simulink model "atrias_system"  (R2014a)
settings: Solver=FixedStepDiscrete  StartTime=0.0  StopTime=inf  FixedStep=sample_time  RelTol=1e-3
PreLoadFcn:
  | set_sampletime
PostLoadFcn:
  | set_sampletime
InitFcn:
  | sys_params
StartFcn:
  | set_sampletime
values from neighbouring files (symbols this model uses):
  A_lpf_velocity = 1 + B1_lpf_velocity + B2_lpf_velocity    [daq_params_osu.m]
  B1_lpf_velocity = -2*exp(-lpf_damping*fcut_velocity*sample_time)*cos(fcut_velocity*sample_time*sqrt(1-lpf_damping^2))    [daq_params_osu.m]
  B2_lpf_velocity = exp(-2*lpf_damping*fcut_velocity*sample_time)    [daq_params_osu.m]
  BOOM_MAX_ENCODER_TICKS = 2^17 - 1    (= 131071)    [daq_params_osu.m]
  BOOM_PITCH_CAL_VALUE_RAD = 0    [daq_params_osu.m]
  BOOM_PITCH_CAL_VALUE_TICKS = 43809    [daq_params_osu.m]
  BOOM_PITCH_ENCODER_RAD_PER_TICK = -2*pi / (2^17 * 2)    (= -2.39684498107e-05)    [daq_params_osu.m]
  BOOM_ROLL_CAL_VALUE_RAD = 0.1271    [daq_params_osu.m]
  BOOM_ROLL_CAL_VALUE_TICKS = 9318    [daq_params_osu.m]
  BOOM_ROLL_ENCODER_RAD_PER_TICK = 2*pi / (2^17 * 7)    (= 6.84812851735e-06)    [daq_params_osu.m]
  BOOM_YAW_ENCODER_RAD_PER_TICK = 2*pi / (2^17 * 9.6)    (= 4.9934270439e-06)    [daq_params_osu.m]
  CURRENT_LIMIT = 100    [daq_params_osu.m]
  fcut_smooth = 16*(2*pi)    (= 100.530964915)    [daq_params_osu.m]
  fcut_unwrap = 8*(2*pi)    (= 50.2654824574)    [daq_params_osu.m]
  gui_disable_cmd = 0    [daq_params_osu.m]
  gui_enable_cmd = 0    [daq_params_osu.m]
  gui_estop_cmd = 0    [daq_params_osu.m]
  gui_reset_cmd = 0    [daq_params_osu.m]
  HIP_ABS_ENCODER_RAD_PER_TICK = 2*pi / 2^13    (= 0.000766990393943)    [daq_params_osu.m]
  HIP_ABS_MAX_ENCODER_TICKS = 2^13 - 1    (= 8191)    [daq_params_osu.m]
  HIP_INC_ENCODER_RAD_PER_TICK = 2*pi / (2500 * 4 * 57)    (= 1.10231321179e-05)    [daq_params_osu.m]
  HIP_INC_MAX_ENCODER_TICKS = 2^16 - 1    (= 65535)    [daq_params_osu.m]
  HIP_MOTOR_CONSTANT = 0.184    [daq_params_osu.m]
  HIP_MTR_GEAR_RATIO = 57    [daq_params_osu.m]
  HIP_MTR_MAX_TORQUE = MTR_HIP_MAX_CURRENT*HIP_MOTOR_CONSTANT*HIP_MTR_GEAR_RATIO    (= 629.28)    [daq_params_osu.m]
  INC_ENC_DIRS = -[ LEG1_MOTOR_A_DIRECTION ... (first row only)    [daq_params_osu.m]
  INC_ENC_RAD_PER_TICK = 2*pi/14000/LEG_MTR_GEAR_RATIO    (= 8.97597901026e-06)    [daq_params_osu.m]
  k_sea = 4118    [sys_params.m]
  LEFT_HIP_CALIB_POS = 0    [daq_params_osu.m]
  LEFT_HIP_CALIB_VAL = 7192 - 2^13    (= -1000)    [daq_params_osu.m]
  LEFT_MOTOR_HIP_DIRECTION = -1.0    (= -1)    [daq_params_osu.m]
  LEG1_LEG_A_CALIB_VAL = 265635200    [daq_params_osu.m]
  LEG1_LEG_A_RAD_PER_CNT = -9.8039216e-09    [daq_params_osu.m]
  LEG1_LEG_B_CALIB_VAL = 174340930    [daq_params_osu.m]
  LEG1_LEG_B_RAD_PER_CNT = -9.8039216e-09    [daq_params_osu.m]
  LEG1_MOTOR_A_DIRECTION = -1.0    (= -1)    [daq_params_osu.m]
  LEG1_MOTOR_B_DIRECTION = -1.0    (= -1)    [daq_params_osu.m]
  LEG1_TRAN_A_CALIB_VAL = 142852340    [daq_params_osu.m]
  LEG1_TRAN_A_RAD_PER_CNT = 9.8039216e-09    [daq_params_osu.m]
  LEG1_TRAN_B_CALIB_VAL = 142241870    [daq_params_osu.m]
  LEG1_TRAN_B_RAD_PER_CNT = -9.8039216e-09    [daq_params_osu.m]
  LEG2_LEG_A_CALIB_VAL = 265322590    [daq_params_osu.m]
  LEG2_LEG_A_RAD_PER_CNT = -9.8039216e-09    [daq_params_osu.m]
  LEG2_LEG_B_CALIB_VAL = 261290850    [daq_params_osu.m]
  LEG2_LEG_B_RAD_PER_CNT = 9.8039216e-09    [daq_params_osu.m]
  LEG2_MOTOR_A_DIRECTION = 1.0    (= 1)    [daq_params_osu.m]
  LEG2_MOTOR_B_DIRECTION = 1.0    (= 1)    [daq_params_osu.m]
  LEG2_TRAN_A_CALIB_VAL = 142172760    [daq_params_osu.m]
  LEG2_TRAN_A_RAD_PER_CNT = 9.8039216e-09    [daq_params_osu.m]
  LEG2_TRAN_B_CALIB_VAL = 142444320    [daq_params_osu.m]
  LEG2_TRAN_B_RAD_PER_CNT = -9.8039216e-09    [daq_params_osu.m]
  LEG_A_CALIB_LOC = pi + 0.305432619099008    (= 3.44702527269)    [daq_params_osu.m]
  LEG_B_CALIB_LOC = pi - 0.305432619099008    (= 2.83616003449)    [daq_params_osu.m]
  LEG_MOTOR_CONSTANT = 0.119    [daq_params_osu.m]
  LEG_MTR_GEAR_RATIO = 50    [daq_params_osu.m]
  LEG_MTR_MAX_TORQUE = MTR_MAX_CURRENT*LEG_MOTOR_CONSTANT*LEG_MTR_GEAR_RATIO    (= 922.25)    [daq_params_osu.m]
  max_encoder_velocity = 200    [daq_params_osu.m]
  MEDULLA_ADC_MAX_VOLTS = 2.70    (= 2.7)    [daq_params_osu.m]
  MEDULLA_ADC_OFFSET_COUNTS = 172    [daq_params_osu.m]
  MEDULLA_STATE_ERROR = 5    [daq_params_osu.m]
  MEDULLA_STATE_HALT = 4    [daq_params_osu.m]
  MEDULLA_STATE_IDLE = 0    [daq_params_osu.m]
  MEDULLA_STATE_RESET = 6    [daq_params_osu.m]
  MEDULLA_STATE_RUN = 2    [daq_params_osu.m]
  MEDULLA_TIMER_FREQ = 32e6    (= 32000000)    [daq_params_osu.m]
  MOTOR_POSITION_LIMITS_LOWER = [2.5; 1.4; 0.4]    [daq_params_osu.m]
  MOTOR_POSITION_LIMITS_UPPER = [4.9; 3.8; 2.5]    [daq_params_osu.m]
  MTR_HIP_MAX_CURRENT = 60.0    (= 60)    [daq_params_osu.m]
  MTR_MAX_CONT_CURRENT = 100.0    (= 100)    [daq_params_osu.m]
  MTR_MAX_COUNT = 19900    [daq_params_osu.m]
  MTR_MAX_CURRENT = 155.0    (= 155)    [daq_params_osu.m]
  nom_sample_time = 0.001    [sys_params.m]
  RIGHT_HIP_CALIB_POS = 0    [daq_params_osu.m]
  RIGHT_HIP_CALIB_VAL = 1091    [daq_params_osu.m]
  RIGHT_MOTOR_HIP_DIRECTION = 1.0    (= 1)    [daq_params_osu.m]
  sample_time = 1/update_freq    (= 0.001)    [daq_params_osu.m]
  sensor_start_time = 8    [daq_params_osu.m]
undefined symbols (not defined in the file or in its folder): max_sensor_velocity
libraries: xpcethercatlib x194, simulink x50, slrtlib x2, dspswit3 x1
(part 2 of 4)

== system atrias_system/DAQ/Elmo Back Left ==
  MotorCmd : Inport
  Constant1 : Constant  Value=4  OutDataTypeStr=Inherit: Inherit via back propagation  SampleTime=-1
  Data Type Conversion124 : DataTypeConversion
  Data Type Conversion125 : DataTypeConversion
  Data Type Conversion126 : DataTypeConversion
  Data Type Conversion2 : DataTypeConversion  OutDataTypeStr=int16
  Drive state transition : Subsystem
  EtherCAT PDO Receive1 : xpcethercatlib/EtherCAT PDO Receive  Priority=2  sig_name=Drive 2 (Elmo Drive).Inputs.Status word  sig_offset=2928  sig_type=uint16  type_size=16  sig_dim=1  device_id=0  sample_time=0.001000
  EtherCAT PDO Receive2 : xpcethercatlib/EtherCAT PDO Receive  Priority=2  sig_name=Drive 2 (Elmo Drive).Inputs.Mode of operation display  sig_offset=2944  sig_type=int8  type_size=8  sig_dim=1  device_id=0  sample_time=0.001000
  "EtherCAT PDO Transmit " : xpcethercatlib/EtherCAT PDO Transmit   Priority=3  sig_name=Drive 2 (Elmo Drive).Outputs.Target Torque  sig_offset=2880  sig_type=int16  type_size=16  sig_dim=1  device_id=0  sample_time=0.001000
  EtherCAT PDO Transmit 1 : xpcethercatlib/EtherCAT PDO Transmit   Priority=3  sig_name=Drive 2 (Elmo Drive).Outputs.Control word  sig_offset=2896  sig_type=uint16  type_size=16  sig_dim=1  device_id=0  sample_time=0.001000
  EtherCAT PDO Transmit 2 : xpcethercatlib/EtherCAT PDO Transmit   Priority=3  sig_name=Drive 2 (Elmo Drive).Outputs.Mode of operation  sig_offset=2912  sig_type=int8  type_size=8  sig_dim=1  device_id=0  sample_time=0.001000
  Mux28 : Mux  Inputs=3
  status : Outport
  wires:
  EtherCAT PDO Receive1/1 -> Drive state transition/1(Status), Data Type Conversion126/1
  EtherCAT PDO Receive2/1 -> Data Type Conversion124/1
  Mux28/1 -> status/1
  Data Type Conversion126/1 -> Mux28/1  "Status Word"
  Data Type Conversion124/1 -> Mux28/2  "Mode of Operation"
  Constant1/1 -> Data Type Conversion125/1
  Drive state transition/1(Control) -> Mux28/3, EtherCAT PDO Transmit 1/1
  Data Type Conversion125/1 -> EtherCAT PDO Transmit 2/1
  MotorCmd/1 -> Data Type Conversion2/1
  Data Type Conversion2/1 -> "EtherCAT PDO Transmit "/1

== system atrias_system/DAQ/Elmo Back Right ==
  MotorCmd : Inport
  Constant1 : Constant  Value=4  OutDataTypeStr=Inherit: Inherit via back propagation  SampleTime=-1
  Data Type Conversion124 : DataTypeConversion
  Data Type Conversion125 : DataTypeConversion
  Data Type Conversion126 : DataTypeConversion
  Data Type Conversion2 : DataTypeConversion  OutDataTypeStr=int16
  Drive state transition : Subsystem
  EtherCAT PDO Receive1 : xpcethercatlib/EtherCAT PDO Receive  Priority=2  sig_name=Drive 9 (Elmo Drive).Inputs.Status word  sig_offset=3168  sig_type=uint16  type_size=16  sig_dim=1  device_id=0  sample_time=0.001000
  EtherCAT PDO Receive2 : xpcethercatlib/EtherCAT PDO Receive  Priority=2  sig_name=Drive 9 (Elmo Drive).Inputs.Mode of operation display  sig_offset=3184  sig_type=int8  type_size=8  sig_dim=1  device_id=0  sample_time=0.001000
  "EtherCAT PDO Transmit " : xpcethercatlib/EtherCAT PDO Transmit   Priority=3  sig_name=Drive 9 (Elmo Drive).Outputs.Target Torque  sig_offset=3120  sig_type=int16  type_size=16  sig_dim=1  device_id=0  sample_time=0.001000
  EtherCAT PDO Transmit 1 : xpcethercatlib/EtherCAT PDO Transmit   Priority=3  sig_name=Drive 9 (Elmo Drive).Outputs.Control word  sig_offset=3136  sig_type=uint16  type_size=16  sig_dim=1  device_id=0  sample_time=0.001000
  EtherCAT PDO Transmit 2 : xpcethercatlib/EtherCAT PDO Transmit   Priority=3  sig_name=Drive 9 (Elmo Drive).Outputs.Mode of operation  sig_offset=3152  sig_type=int8  type_size=8  sig_dim=1  device_id=0  sample_time=0.001000
  Mux28 : Mux  Inputs=3
  status : Outport
  wires:
  EtherCAT PDO Receive1/1 -> Drive state transition/1(Status), Data Type Conversion126/1
  EtherCAT PDO Receive2/1 -> Data Type Conversion124/1
  Mux28/1 -> status/1
  Data Type Conversion126/1 -> Mux28/1  "Status Word"
  Data Type Conversion124/1 -> Mux28/2  "Mode of Operation"
  Constant1/1 -> Data Type Conversion125/1
  Drive state transition/1(Control) -> Mux28/3, EtherCAT PDO Transmit 1/1
  Data Type Conversion125/1 -> EtherCAT PDO Transmit 2/1
  MotorCmd/1 -> Data Type Conversion2/1
  Data Type Conversion2/1 -> "EtherCAT PDO Transmit "/1

== system atrias_system/DAQ/Elmo Front Left ==
  MotorCmd : Inport
  Constant1 : Constant  Value=4  OutDataTypeStr=Inherit: Inherit via back propagation  SampleTime=-1
  Data Type Conversion124 : DataTypeConversion
  Data Type Conversion125 : DataTypeConversion
  Data Type Conversion126 : DataTypeConversion
  Data Type Conversion2 : DataTypeConversion  OutDataTypeStr=int16
  Drive state transition : Subsystem
  EtherCAT PDO Receive1 : xpcethercatlib/EtherCAT PDO Receive  Priority=2  sig_name=Drive 3 (Elmo Drive).Inputs.Status word  sig_offset=3008  sig_type=uint16  type_size=16  sig_dim=1  device_id=0  sample_time=0.001000
  EtherCAT PDO Receive2 : xpcethercatlib/EtherCAT PDO Receive  Priority=2  sig_name=Drive 3 (Elmo Drive).Inputs.Mode of operation display  sig_offset=3024  sig_type=int8  type_size=8  sig_dim=1  device_id=0  sample_time=0.001000
  "EtherCAT PDO Transmit " : xpcethercatlib/EtherCAT PDO Transmit   Priority=3  sig_name=Drive 3 (Elmo Drive).Outputs.Target Torque  sig_offset=2960  sig_type=int16  type_size=16  sig_dim=1  device_id=0  sample_time=0.001000
  EtherCAT PDO Transmit 1 : xpcethercatlib/EtherCAT PDO Transmit   Priority=3  sig_name=Drive 3 (Elmo Drive).Outputs.Control word  sig_offset=2976  sig_type=uint16  type_size=16  sig_dim=1  device_id=0  sample_time=0.001000
  EtherCAT PDO Transmit 2 : xpcethercatlib/EtherCAT PDO Transmit   Priority=3  sig_name=Drive 3 (Elmo Drive).Outputs.Mode of operation  sig_offset=2992  sig_type=int8  type_size=8  sig_dim=1  device_id=0  sample_time=0.001000
  Mux28 : Mux  Inputs=3
  status : Outport
  wires:
  EtherCAT PDO Receive1/1 -> Drive state transition/1(Status), Data Type Conversion126/1
  EtherCAT PDO Receive2/1 -> Data Type Conversion124/1
  Mux28/1 -> status/1
  Data Type Conversion126/1 -> Mux28/1  "Status Word"
  Data Type Conversion124/1 -> Mux28/2  "Mode of Operation"
  Constant1/1 -> Data Type Conversion125/1
  Drive state transition/1(Control) -> Mux28/3, EtherCAT PDO Transmit 1/1
  Data Type Conversion125/1 -> EtherCAT PDO Transmit 2/1
  MotorCmd/1 -> Data Type Conversion2/1
  Data Type Conversion2/1 -> "EtherCAT PDO Transmit "/1

== system atrias_system/DAQ/Elmo Front Right ==
  MotorCmd : Inport
  Constant1 : Constant  Value=4  OutDataTypeStr=Inherit: Inherit via back propagation  SampleTime=-1
  Data Type Conversion124 : DataTypeConversion
  Data Type Conversion125 : DataTypeConversion
  Data Type Conversion126 : DataTypeConversion
  Data Type Conversion2 : DataTypeConversion  OutDataTypeStr=int16
  Drive state transition : Subsystem
  EtherCAT PDO Receive1 : xpcethercatlib/EtherCAT PDO Receive  Priority=2  sig_name=Drive 8 (Elmo Drive).Inputs.Status word  sig_offset=3088  sig_type=uint16  type_size=16  sig_dim=1  device_id=0  sample_time=0.001000
  EtherCAT PDO Receive2 : xpcethercatlib/EtherCAT PDO Receive  Priority=2  sig_name=Drive 8 (Elmo Drive).Inputs.Mode of operation display  sig_offset=3104  sig_type=int8  type_size=8  sig_dim=1  device_id=0  sample_time=0.001000
  "EtherCAT PDO Transmit " : xpcethercatlib/EtherCAT PDO Transmit   Priority=3  sig_name=Drive 8 (Elmo Drive).Outputs.Target Torque  sig_offset=3040  sig_type=int16  type_size=16  sig_dim=1  device_id=0  sample_time=0.001000
  EtherCAT PDO Transmit 1 : xpcethercatlib/EtherCAT PDO Transmit   Priority=3  sig_name=Drive 8 (Elmo Drive).Outputs.Control word  sig_offset=3056  sig_type=uint16  type_size=16  sig_dim=1  device_id=0  sample_time=0.001000
  EtherCAT PDO Transmit 2 : xpcethercatlib/EtherCAT PDO Transmit   Priority=3  sig_name=Drive 8 (Elmo Drive).Outputs.Mode of operation  sig_offset=3072  sig_type=int8  type_size=8  sig_dim=1  device_id=0  sample_time=0.001000
  Mux28 : Mux  Inputs=3
  status : Outport
  wires:
  EtherCAT PDO Receive1/1 -> Drive state transition/1(Status), Data Type Conversion126/1
  EtherCAT PDO Receive2/1 -> Data Type Conversion124/1
  Mux28/1 -> status/1
  Data Type Conversion126/1 -> Mux28/1  "Status Word"
  Data Type Conversion124/1 -> Mux28/2  "Mode of Operation"
  Constant1/1 -> Data Type Conversion125/1
  Drive state transition/1(Control) -> Mux28/3, EtherCAT PDO Transmit 1/1
  Data Type Conversion125/1 -> EtherCAT PDO Transmit 2/1
  MotorCmd/1 -> Data Type Conversion2/1
  Data Type Conversion2/1 -> "EtherCAT PDO Transmit "/1

== system atrias_system/DAQ/Fail Safe ==
  note: any of the absolute leg encoders read zero?
  note: all encoders read zero?
  note: any of the absolute lateral encdoers read all
      | zeros/ones in the first 10 readings?
  encoder signals : Inport
  Clock : Clock
  Compare To Constant : simulink/Logic and Bit Operations/Compare To Constant  relop===  const=2^13-1  OutDataTypeStr=boolean
  Compare To Zero : simulink/Logic and Bit Operations/Compare To Zero  relop===  OutDataTypeStr=boolean
  Compare To Zero1 : simulink/Logic and Bit Operations/Compare To Zero  relop===  OutDataTypeStr=boolean
  Compare To Zero2 : simulink/Logic and Bit Operations/Compare To Zero  relop===  OutDataTypeStr=boolean
  Data Type Conversion : DataTypeConversion  OutDataTypeStr=boolean
  Data Type Conversion1 : DataTypeConversion  OutDataTypeStr=boolean
  Data Type Conversion2 : DataTypeConversion  OutDataTypeStr=uint8
  Data Type Conversion3 : DataTypeConversion  OutDataTypeStr=uint8
  Initial Sensor Reading : simulink/Logic and Bit Operations/Compare To Constant  relop=<=  const=sensor_start_time+10*sample_time  OutDataTypeStr=boolean
  Logical Operator{,1,3..4} (4 alike) : Logic  AllPortsSameDT=off  OutDataTypeStr=boolean
  Logical Operator2 : Logic  Operator=OR  Inputs=3  AllPortsSameDT=off  OutDataTypeStr=boolean
  LogicalOperator5 : Logic  Operator=OR  AllPortsSameDT=off  OutDataTypeStr=boolean
  Sensors Active : simulink/Logic and Bit Operations/Compare To Constant  relop=>=  const=sensor_start_time  OutDataTypeStr=boolean
  Sum of Elements : Sum  Inputs=+
  Sum of Elements1 : Sum  Inputs=+
  Sum of Elements2 : Sum  Inputs=+
  absolute lateral encoders : Selector  InputPortWidth=15  Indices=[9 11]
  absolute leg encoders : Selector  InputPortWidth=15  Indices=[1 2 3 4 5 6 7 8]
  stop? : Outport
  wires:
  LogicalOperator5/1 -> Logical Operator3/2
  Compare To Constant/1 -> LogicalOperator5/2
  Compare To Zero2/1 -> LogicalOperator5/1
  absolute leg encoders/1 -> Compare To Zero1/1
  Compare To Zero1/1 -> Logical Operator1/2
  Logical Operator2/1 -> stop?/1
  Logical Operator1/1 -> Data Type Conversion2/1
  Compare To Zero/1 -> Logical Operator/1
  encoder signals/1 -> absolute lateral encoders/1, absolute leg encoders/1, Sum of Elements/1
  Logical Operator/1 -> Logical Operator2/1
  Sum of Elements/1 -> Compare To Zero/1
  Sensors Active/1 -> Logical Operator4/1, Logical Operator/2, Logical Operator1/1
  absolute lateral encoders/1 -> Compare To Zero2/1, Compare To Constant/1
  Clock/1 -> Initial Sensor Reading/1, Sensors Active/1
  Initial Sensor Reading/1 -> Logical Operator4/2
  Logical Operator4/1 -> Logical Operator3/1
  Logical Operator3/1 -> Data Type Conversion3/1
  Sum of Elements1/1 -> Data Type Conversion/1
  Sum of Elements2/1 -> Data Type Conversion1/1
  Data Type Conversion/1 -> Logical Operator2/3
  Data Type Conversion1/1 -> Logical Operator2/2
  Data Type Conversion2/1 -> Sum of Elements2/1
  Data Type Conversion3/1 -> Sum of Elements1/1

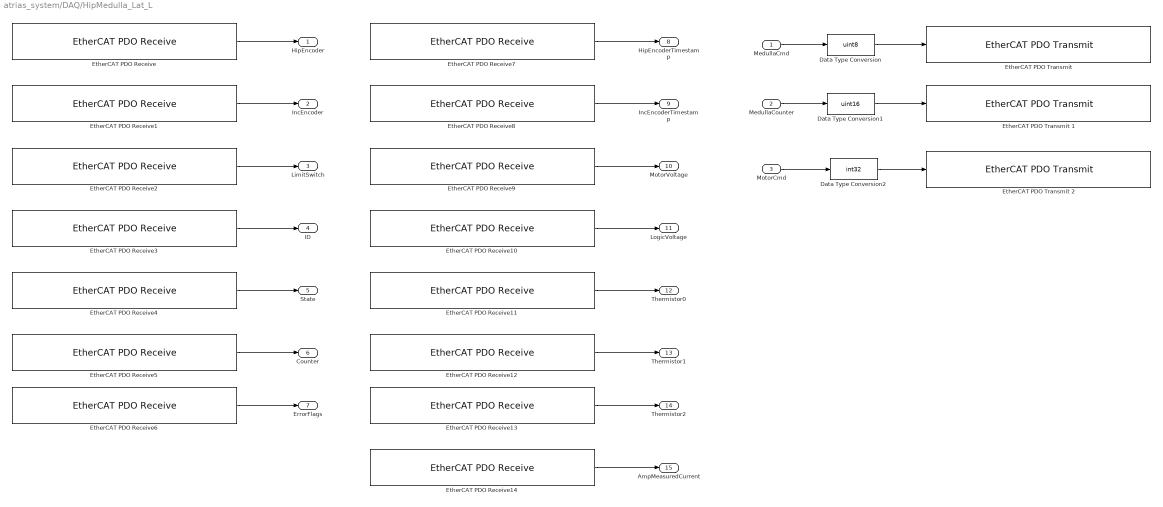
== system atrias_system/DAQ/HipMedulla_Lat_L ==
  MedullaCmd : Inport
  MedullaCounter : Inport  Port=2
  MotorCmd : Inport  Port=3
  Data Type Conversion : DataTypeConversion  OutDataTypeStr=uint8
  Data Type Conversion1 : DataTypeConversion  OutDataTypeStr=uint16
  Data Type Conversion2 : DataTypeConversion  OutDataTypeStr=int32
  EtherCAT PDO Receive : xpcethercatlib/EtherCAT PDO Receive  Priority=2  sig_name=Box 1 (ATRIAS 2.1 Hip (Medulla 1.5)).Hip Encoder.Encoder  sig_offset=632  sig_type=uint32  type_size=32  sig_dim=1  device_id=0  sample_time=0.001000
  EtherCAT PDO Receive1 : xpcethercatlib/EtherCAT PDO Receive  Priority=2  sig_name=Box 1 (ATRIAS 2.1 Hip (Medulla 1.5)).Incremental Encoder.Incremental Encoder  sig_offset=776  sig_type=uint16  type_size=16  sig_dim=1  device_id=0  sample_time=0.001000
  EtherCAT PDO Receive10 : xpcethercatlib/EtherCAT PDO Receive  Priority=2  sig_name=Box 1 (ATRIAS 2.1 Hip (Medulla 1.5)).Power.Logic Voltage  sig_offset=696  sig_type=uint16  type_size=16  sig_dim=1  device_id=0  sample_time=0.001000
  EtherCAT PDO Receive11 : xpcethercatlib/EtherCAT PDO Receive  Priority=2  sig_name=Box 1 (ATRIAS 2.1 Hip (Medulla 1.5)).Thermistors.Thermistor 0  sig_offset=712  sig_type=uint16  type_size=16  sig_dim=1  device_id=0  sample_time=0.001000
  EtherCAT PDO Receive12 : xpcethercatlib/EtherCAT PDO Receive  Priority=2  sig_name=Box 1 (ATRIAS 2.1 Hip (Medulla 1.5)).Thermistors.Thermistor 1  sig_offset=728  sig_type=uint16  type_size=16  sig_dim=1  device_id=0  sample_time=0.001000
  EtherCAT PDO Receive13 : xpcethercatlib/EtherCAT PDO Receive  Priority=2  sig_name=Box 1 (ATRIAS 2.1 Hip (Medulla 1.5)).Thermistors.Thermistor 2  sig_offset=744  sig_type=uint16  type_size=16  sig_dim=1  device_id=0  sample_time=0.001000
  EtherCAT PDO Receive14 : xpcethercatlib/EtherCAT PDO Receive  Priority=2  sig_name=Box 1 (ATRIAS 2.1 Hip (Medulla 1.5)).Measured Current.Amp Measured Current  sig_offset=760  sig_type=int16  type_size=16  sig_dim=1  device_id=0  sample_time=0.001000
  EtherCAT PDO Receive2 : xpcethercatlib/EtherCAT PDO Receive  Priority=2  sig_name=Box 1 (ATRIAS 2.1 Hip (Medulla 1.5)).uController Status.Limit Switch  sig_offset=624  sig_type=uint8  type_size=8  sig_dim=1  device_id=0  sample_time=0.001000
  EtherCAT PDO Receive3 : xpcethercatlib/EtherCAT PDO Receive  Priority=2  sig_name=Box 1 (ATRIAS 2.1 Hip (Medulla 1.5)).uController Status.ID  sig_offset=592  sig_type=uint8  type_size=8  sig_dim=1  device_id=0  sample_time=0.001000
  EtherCAT PDO Receive4 : xpcethercatlib/EtherCAT PDO Receive  Priority=2  sig_name=Box 1 (ATRIAS 2.1 Hip (Medulla 1.5)).uController Status.State  sig_offset=600  sig_type=uint8  type_size=8  sig_dim=1  device_id=0  sample_time=0.001000
  EtherCAT PDO Receive5 : xpcethercatlib/EtherCAT PDO Receive  Priority=2  sig_name=Box 1 (ATRIAS 2.1 Hip (Medulla 1.5)).uController Status.Counter  sig_offset=608  sig_type=uint8  type_size=8  sig_dim=1  device_id=0  sample_time=0.001000
  EtherCAT PDO Receive6 : xpcethercatlib/EtherCAT PDO Receive  Priority=2  sig_name=Box 1 (ATRIAS 2.1 Hip (Medulla 1.5)).uController Status.Error Flags  sig_offset=616  sig_type=uint8  type_size=8  sig_dim=1  device_id=0  sample_time=0.001000
  EtherCAT PDO Receive7 : xpcethercatlib/EtherCAT PDO Receive  Priority=2  sig_name=Box 1 (ATRIAS 2.1 Hip (Medulla 1.5)).Hip Encoder.Timestamp  sig_offset=664  sig_type=uint16  type_size=16  sig_dim=1  device_id=0  sample_time=0.001000
  EtherCAT PDO Receive8 : xpcethercatlib/EtherCAT PDO Receive  Priority=2  sig_name=Box 1 (ATRIAS 2.1 Hip (Medulla 1.5)).Incremental Encoder.Incremental Encoder Timestamp  sig_offset=792  sig_type=uint16  type_size=16  sig_dim=1  device_id=0  sample_time=0.001000
  EtherCAT PDO Receive9 : xpcethercatlib/EtherCAT PDO Receive  Priority=2  sig_name=Box 1 (ATRIAS 2.1 Hip (Medulla 1.5)).Power.Motor Voltage  sig_offset=680  sig_type=uint16  type_size=16  sig_dim=1  device_id=0  sample_time=0.001000
  "EtherCAT PDO Transmit " : xpcethercatlib/EtherCAT PDO Transmit   Priority=3  sig_name=Box 1 (ATRIAS 2.1 Hip (Medulla 1.5)).uControllerInput.Command  sig_offset=592  sig_type=uint8  type_size=8  sig_dim=1  device_id=0  sample_time=0.001000
  EtherCAT PDO Transmit 1 : xpcethercatlib/EtherCAT PDO Transmit   Priority=3  sig_name=Box 1 (ATRIAS 2.1 Hip (Medulla 1.5)).uControllerInput.Counter  sig_offset=600  sig_type=uint16  type_size=16  sig_dim=1  device_id=0  sample_time=0.001000
  EtherCAT PDO Transmit 2 : xpcethercatlib/EtherCAT PDO Transmit   Priority=3  sig_name=Box 1 (ATRIAS 2.1 Hip (Medulla 1.5)).uControllerInput.Motor Current  sig_offset=616  sig_type=int32  type_size=32  sig_dim=1  device_id=0  sample_time=0.001000
  HipEncoder : Outport
  IncEncoder : Outport  Port=2
  LimitSwitch : Outport  Port=3
  ID : Outport  Port=4
  State : Outport  Port=5
  Counter : Outport  Port=6
  ErrorFlags : Outport  Port=7
  HipEncoderTimestamp : Outport  Port=8
  IncEncoderTimestamp : Outport  Port=9
  MotorVoltage : Outport  Port=10
  LogicVoltage : Outport  Port=11
  Thermistor0 : Outport  Port=12
  Thermistor1 : Outport  Port=13
  Thermistor2 : Outport  Port=14
  AmpMeasuredCurrent : Outport  Port=15
  wires:
  Data Type Conversion/1 -> "EtherCAT PDO Transmit "/1
  Data Type Conversion1/1 -> EtherCAT PDO Transmit 1/1
  Data Type Conversion2/1 -> EtherCAT PDO Transmit 2/1
  MedullaCmd/1 -> Data Type Conversion/1
  MedullaCounter/1 -> Data Type Conversion1/1
  MotorCmd/1 -> Data Type Conversion2/1
  EtherCAT PDO Receive8/1 -> IncEncoderTimestamp/1
  EtherCAT PDO Receive/1 -> HipEncoder/1
  EtherCAT PDO Receive7/1 -> HipEncoderTimestamp/1
  EtherCAT PDO Receive1/1 -> IncEncoder/1
  EtherCAT PDO Receive5/1 -> Counter/1
  EtherCAT PDO Receive3/1 -> ID/1
  EtherCAT PDO Receive2/1 -> LimitSwitch/1
  EtherCAT PDO Receive4/1 -> State/1
  EtherCAT PDO Receive6/1 -> ErrorFlags/1
  EtherCAT PDO Receive10/1 -> LogicVoltage/1
  EtherCAT PDO Receive9/1 -> MotorVoltage/1
  EtherCAT PDO Receive11/1 -> Thermistor0/1
  EtherCAT PDO Receive12/1 -> Thermistor1/1
  EtherCAT PDO Receive13/1 -> Thermistor2/1
  EtherCAT PDO Receive14/1 -> AmpMeasuredCurrent/1

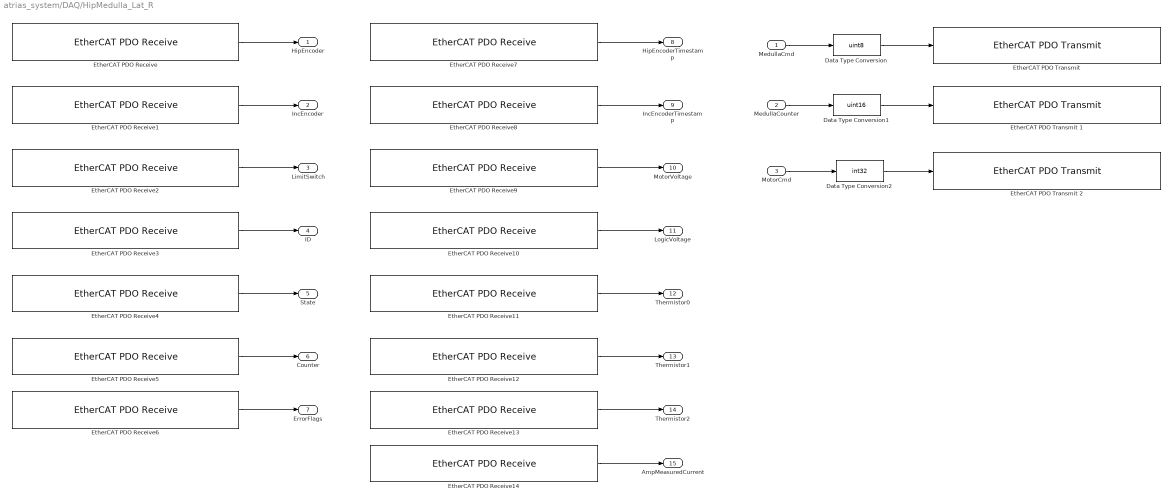
== system atrias_system/DAQ/HipMedulla_Lat_R ==
  MedullaCmd : Inport
  MedullaCounter : Inport  Port=2
  MotorCmd : Inport  Port=3
  Data Type Conversion : DataTypeConversion  OutDataTypeStr=uint8
  Data Type Conversion1 : DataTypeConversion  OutDataTypeStr=uint16
  Data Type Conversion2 : DataTypeConversion  OutDataTypeStr=int32
  EtherCAT PDO Receive : xpcethercatlib/EtherCAT PDO Receive  Priority=2  sig_name=Box 10 (ATRIAS 2.1 Hip (Medulla 1.5)).Hip Encoder.Encoder  sig_offset=2384  sig_type=uint32  type_size=32  sig_dim=1  device_id=0  sample_time=0.001000
  EtherCAT PDO Receive1 : xpcethercatlib/EtherCAT PDO Receive  Priority=2  sig_name=Box 10 (ATRIAS 2.1 Hip (Medulla 1.5)).Incremental Encoder.Incremental Encoder  sig_offset=2528  sig_type=uint16  type_size=16  sig_dim=1  device_id=0  sample_time=0.001000
  EtherCAT PDO Receive10 : xpcethercatlib/EtherCAT PDO Receive  Priority=2  sig_name=Box 10 (ATRIAS 2.1 Hip (Medulla 1.5)).Power.Logic Voltage  sig_offset=2448  sig_type=uint16  type_size=16  sig_dim=1  device_id=0  sample_time=0.001000
  EtherCAT PDO Receive11 : xpcethercatlib/EtherCAT PDO Receive  Priority=2  sig_name=Box 10 (ATRIAS 2.1 Hip (Medulla 1.5)).Thermistors.Thermistor 0  sig_offset=2464  sig_type=uint16  type_size=16  sig_dim=1  device_id=0  sample_time=0.001000
  EtherCAT PDO Receive12 : xpcethercatlib/EtherCAT PDO Receive  Priority=2  sig_name=Box 10 (ATRIAS 2.1 Hip (Medulla 1.5)).Thermistors.Thermistor 1  sig_offset=2480  sig_type=uint16  type_size=16  sig_dim=1  device_id=0  sample_time=0.001000
  EtherCAT PDO Receive13 : xpcethercatlib/EtherCAT PDO Receive  Priority=2  sig_name=Box 10 (ATRIAS 2.1 Hip (Medulla 1.5)).Thermistors.Thermistor 2  sig_offset=2496  sig_type=uint16  type_size=16  sig_dim=1  device_id=0  sample_time=0.001000
  EtherCAT PDO Receive14 : xpcethercatlib/EtherCAT PDO Receive  Priority=2  sig_name=Box 10 (ATRIAS 2.1 Hip (Medulla 1.5)).Measured Current.Amp Measured Current  sig_offset=2512  sig_type=int16  type_size=16  sig_dim=1  device_id=0  sample_time=0.001000
  EtherCAT PDO Receive2 : xpcethercatlib/EtherCAT PDO Receive  Priority=2  sig_name=Box 10 (ATRIAS 2.1 Hip (Medulla 1.5)).uController Status.Limit Switch  sig_offset=2376  sig_type=uint8  type_size=8  sig_dim=1  device_id=0  sample_time=0.001000
  EtherCAT PDO Receive3 : xpcethercatlib/EtherCAT PDO Receive  Priority=2  sig_name=Box 10 (ATRIAS 2.1 Hip (Medulla 1.5)).uController Status.ID  sig_offset=2344  sig_type=uint8  type_size=8  sig_dim=1  device_id=0  sample_time=0.001000
  EtherCAT PDO Receive4 : xpcethercatlib/EtherCAT PDO Receive  Priority=2  sig_name=Box 10 (ATRIAS 2.1 Hip (Medulla 1.5)).uController Status.State  sig_offset=2352  sig_type=uint8  type_size=8  sig_dim=1  device_id=0  sample_time=0.001000
  EtherCAT PDO Receive5 : xpcethercatlib/EtherCAT PDO Receive  Priority=2  sig_name=Box 10 (ATRIAS 2.1 Hip (Medulla 1.5)).uController Status.Counter  sig_offset=2360  sig_type=uint8  type_size=8  sig_dim=1  device_id=0  sample_time=0.001000
  EtherCAT PDO Receive6 : xpcethercatlib/EtherCAT PDO Receive  Priority=2  sig_name=Box 10 (ATRIAS 2.1 Hip (Medulla 1.5)).uController Status.Error Flags  sig_offset=2368  sig_type=uint8  type_size=8  sig_dim=1  device_id=0  sample_time=0.001000
  EtherCAT PDO Receive7 : xpcethercatlib/EtherCAT PDO Receive  Priority=2  sig_name=Box 10 (ATRIAS 2.1 Hip (Medulla 1.5)).Hip Encoder.Timestamp  sig_offset=2416  sig_type=uint16  type_size=16  sig_dim=1  device_id=0  sample_time=0.001000
  EtherCAT PDO Receive8 : xpcethercatlib/EtherCAT PDO Receive  Priority=2  sig_name=Box 10 (ATRIAS 2.1 Hip (Medulla 1.5)).Incremental Encoder.Incremental Encoder Timestamp  sig_offset=2544  sig_type=uint16  type_size=16  sig_dim=1  device_id=0  sample_time=0.001000
  EtherCAT PDO Receive9 : xpcethercatlib/EtherCAT PDO Receive  Priority=2  sig_name=Box 10 (ATRIAS 2.1 Hip (Medulla 1.5)).Power.Motor Voltage  sig_offset=2432  sig_type=uint16  type_size=16  sig_dim=1  device_id=0  sample_time=0.001000
  EtherCAT PDO Transmit : xpcethercatlib/EtherCAT PDO Transmit   Priority=3  sig_name=Box 10 (ATRIAS 2.1 Hip (Medulla 1.5)).uControllerInput.Command  sig_offset=2344  sig_type=uint8  type_size=8  sig_dim=1  device_id=0  sample_time=0.001000
  "EtherCAT PDO Transmit 1 " : xpcethercatlib/EtherCAT PDO Transmit   Priority=3  sig_name=Box 10 (ATRIAS 2.1 Hip (Medulla 1.5)).uControllerInput.Counter  sig_offset=2352  sig_type=uint16  type_size=16  sig_dim=1  device_id=0  sample_time=0.001000
  EtherCAT PDO Transmit 2 : xpcethercatlib/EtherCAT PDO Transmit   Priority=3  sig_name=Box 10 (ATRIAS 2.1 Hip (Medulla 1.5)).uControllerInput.Motor Current  sig_offset=2368  sig_type=int32  type_size=32  sig_dim=1  device_id=0  sample_time=0.001000
  HipEncoder : Outport
  IncEncoder : Outport  Port=2
  LimitSwitch : Outport  Port=3
  ID : Outport  Port=4
  State : Outport  Port=5
  Counter : Outport  Port=6
  ErrorFlags : Outport  Port=7
  HipEncoderTimestamp : Outport  Port=8
  IncEncoderTimestamp : Outport  Port=9
  MotorVoltage : Outport  Port=10
  LogicVoltage : Outport  Port=11
  Thermistor0 : Outport  Port=12
  Thermistor1 : Outport  Port=13
  Thermistor2 : Outport  Port=14
  AmpMeasuredCurrent : Outport  Port=15
  wires:
  Data Type Conversion/1 -> EtherCAT PDO Transmit/1
  Data Type Conversion1/1 -> "EtherCAT PDO Transmit 1 "/1
  Data Type Conversion2/1 -> EtherCAT PDO Transmit 2/1
  MedullaCmd/1 -> Data Type Conversion/1
  MedullaCounter/1 -> Data Type Conversion1/1
  MotorCmd/1 -> Data Type Conversion2/1
  EtherCAT PDO Receive8/1 -> IncEncoderTimestamp/1
  EtherCAT PDO Receive/1 -> HipEncoder/1
  EtherCAT PDO Receive7/1 -> HipEncoderTimestamp/1
  EtherCAT PDO Receive1/1 -> IncEncoder/1
  EtherCAT PDO Receive5/1 -> Counter/1
  EtherCAT PDO Receive3/1 -> ID/1
  EtherCAT PDO Receive2/1 -> LimitSwitch/1
  EtherCAT PDO Receive4/1 -> State/1
  EtherCAT PDO Receive6/1 -> ErrorFlags/1
  EtherCAT PDO Receive10/1 -> LogicVoltage/1
  EtherCAT PDO Receive9/1 -> MotorVoltage/1
  EtherCAT PDO Receive11/1 -> Thermistor0/1
  EtherCAT PDO Receive12/1 -> Thermistor1/1
  EtherCAT PDO Receive13/1 -> Thermistor2/1
  EtherCAT PDO Receive14/1 -> AmpMeasuredCurrent/1

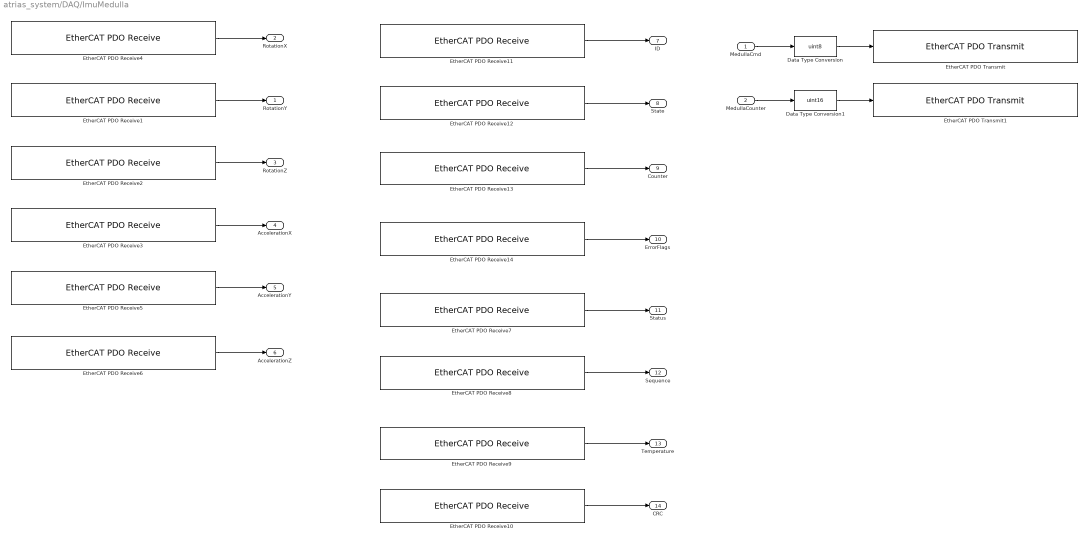
== system atrias_system/DAQ/ImuMedulla ==
  MedullaCmd : Inport
  MedullaCounter : Inport  Port=2
  Data Type Conversion : DataTypeConversion  OutDataTypeStr=uint8
  Data Type Conversion1 : DataTypeConversion  OutDataTypeStr=uint16
  EtherCAT PDO Receive1 : xpcethercatlib/EtherCAT PDO Receive  Priority=2  sig_name=Box 7 (ATRIAS 2.1 IMU (Medulla 1.5)).Rotation.Y  sig_offset=2464  sig_type=single  type_size=32  sig_dim=1  device_id=0  sample_time=0.001000
  EtherCAT PDO Receive10 : xpcethercatlib/EtherCAT PDO Receive  Priority=2  sig_name=Box 7 (ATRIAS 2.1 IMU (Medulla 1.5)).Status.CRC  sig_offset=2656  sig_type=uint32  type_size=32  sig_dim=1  device_id=0  sample_time=0.001000
  EtherCAT PDO Receive11 : xpcethercatlib/EtherCAT PDO Receive  Priority=2  sig_name=Box 7 (ATRIAS 2.1 IMU (Medulla 1.5)).uController Status.ID  sig_offset=2400  sig_type=uint8  type_size=8  sig_dim=1  device_id=0  sample_time=0.001000
  EtherCAT PDO Receive12 : xpcethercatlib/EtherCAT PDO Receive  Priority=2  sig_name=Box 7 (ATRIAS 2.1 IMU (Medulla 1.5)).uController Status.State  sig_offset=2408  sig_type=uint8  type_size=8  sig_dim=1  device_id=0  sample_time=0.001000
  EtherCAT PDO Receive13 : xpcethercatlib/EtherCAT PDO Receive  Priority=2  sig_name=Box 7 (ATRIAS 2.1 IMU (Medulla 1.5)).uController Status.Counter  sig_offset=2416  sig_type=uint8  type_size=8  sig_dim=1  device_id=0  sample_time=0.001000
  EtherCAT PDO Receive14 : xpcethercatlib/EtherCAT PDO Receive  Priority=2  sig_name=Box 8 (ATRIAS 2.1 Boom (Medulla 1.5)).uController Status.Error Flags  sig_offset=2712  sig_type=uint8  type_size=8  sig_dim=1  device_id=0  sample_time=0.001000
  EtherCAT PDO Receive2 : xpcethercatlib/EtherCAT PDO Receive  Priority=2  sig_name=Box 7 (ATRIAS 2.1 IMU (Medulla 1.5)).Rotation.Z  sig_offset=2496  sig_type=single  type_size=32  sig_dim=1  device_id=0  sample_time=0.001000
  EtherCAT PDO Receive3 : xpcethercatlib/EtherCAT PDO Receive  Priority=2  sig_name=Box 7 (ATRIAS 2.1 IMU (Medulla 1.5)).Acceleration.X  sig_offset=2528  sig_type=single  type_size=32  sig_dim=1  device_id=0  sample_time=0.001000
  EtherCAT PDO Receive4 : xpcethercatlib/EtherCAT PDO Receive  Priority=2  sig_name=Box 7 (ATRIAS 2.1 IMU (Medulla 1.5)).Rotation.X  sig_offset=2432  sig_type=single  type_size=32  sig_dim=1  device_id=0  sample_time=0.001000
  EtherCAT PDO Receive5 : xpcethercatlib/EtherCAT PDO Receive  Priority=2  sig_name=Box 7 (ATRIAS 2.1 IMU (Medulla 1.5)).Acceleration.Y  sig_offset=2560  sig_type=single  type_size=32  sig_dim=1  device_id=0  sample_time=0.001000
  EtherCAT PDO Receive6 : xpcethercatlib/EtherCAT PDO Receive  Priority=2  sig_name=Box 7 (ATRIAS 2.1 IMU (Medulla 1.5)).Acceleration.Z  sig_offset=2592  sig_type=single  type_size=32  sig_dim=1  device_id=0  sample_time=0.001000
  EtherCAT PDO Receive7 : xpcethercatlib/EtherCAT PDO Receive  Priority=2  sig_name=Box 7 (ATRIAS 2.1 IMU (Medulla 1.5)).Status.Status  sig_offset=2624  sig_type=uint8  type_size=8  sig_dim=1  device_id=0  sample_time=0.001000
  EtherCAT PDO Receive8 : xpcethercatlib/EtherCAT PDO Receive  Priority=2  sig_name=Box 7 (ATRIAS 2.1 IMU (Medulla 1.5)).Status.Sequence  sig_offset=2632  sig_type=uint8  type_size=8  sig_dim=1  device_id=0  sample_time=0.001000
  EtherCAT PDO Receive9 : xpcethercatlib/EtherCAT PDO Receive  Priority=2  sig_name=Box 7 (ATRIAS 2.1 IMU (Medulla 1.5)).Status.Temperature  sig_offset=2640  sig_type=int16  type_size=16  sig_dim=1  device_id=0  sample_time=0.001000
  EtherCAT PDO Transmit : xpcethercatlib/EtherCAT PDO Transmit   Priority=3  sig_name=Box 7 (ATRIAS 2.1 IMU (Medulla 1.5)).uControllerInput.Command  sig_offset=2400  sig_type=uint8  type_size=8  sig_dim=1  device_id=0  sample_time=0.001000
  EtherCAT PDO Transmit1 : xpcethercatlib/EtherCAT PDO Transmit   Priority=3  sig_name=Box 7 (ATRIAS 2.1 IMU (Medulla 1.5)).uControllerInput.Counter  sig_offset=2408  sig_type=uint16  type_size=16  sig_dim=1  device_id=0  sample_time=0.001000
  RotationY : Outport
  RotationX : Outport  Port=2
  RotationZ : Outport  Port=3
  AccelerationX : Outport  Port=4
  AccelerationY : Outport  Port=5
  AccelerationZ : Outport  Port=6
  ID : Outport  Port=7
  State : Outport  Port=8
  Counter : Outport  Port=9
  ErrorFlags : Outport  Port=10
  Status : Outport  Port=11
  Sequence : Outport  Port=12
  Temperature : Outport  Port=13
  CRC : Outport  Port=14
  wires:
  EtherCAT PDO Receive11/1 -> ID/1
  EtherCAT PDO Receive10/1 -> CRC/1
  EtherCAT PDO Receive9/1 -> Temperature/1
  EtherCAT PDO Receive8/1 -> Sequence/1
  EtherCAT PDO Receive7/1 -> Status/1
  EtherCAT PDO Receive6/1 -> AccelerationZ/1
  EtherCAT PDO Receive5/1 -> AccelerationY/1
  EtherCAT PDO Receive3/1 -> AccelerationX/1
  EtherCAT PDO Receive2/1 -> RotationZ/1
  EtherCAT PDO Receive1/1 -> RotationY/1
  EtherCAT PDO Receive4/1 -> RotationX/1
  MedullaCounter/1 -> Data Type Conversion1/1
  MedullaCmd/1 -> Data Type Conversion/1
  Data Type Conversion1/1 -> EtherCAT PDO Transmit1/1
  Data Type Conversion/1 -> EtherCAT PDO Transmit/1
  EtherCAT PDO Receive12/1 -> State/1
  EtherCAT PDO Receive13/1 -> Counter/1
  EtherCAT PDO Receive14/1 -> ErrorFlags/1

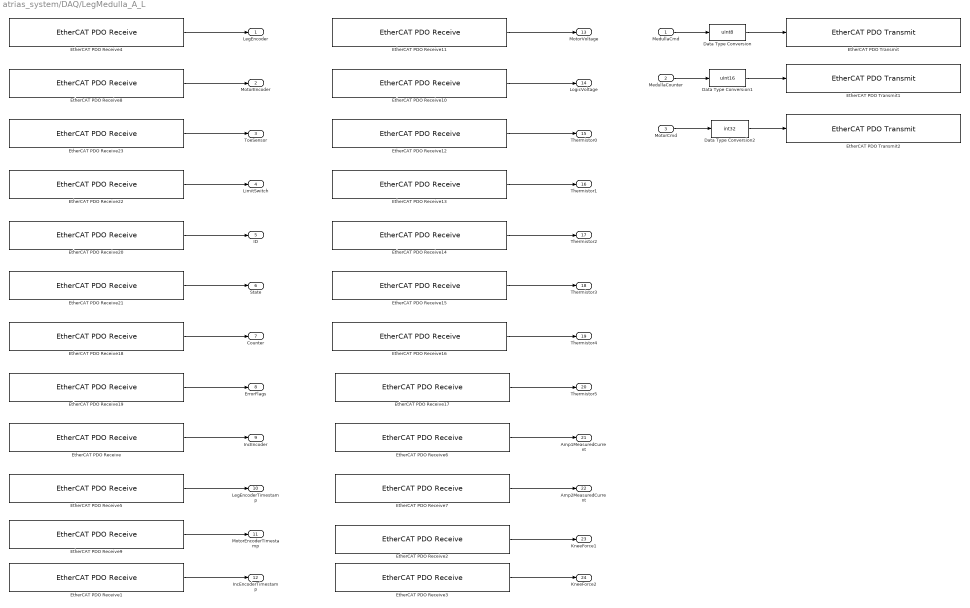
== system atrias_system/DAQ/LegMedulla_A_L ==
  MedullaCmd : Inport
  MedullaCounter : Inport  Port=2
  MotorCmd : Inport  Port=3
  Data Type Conversion : DataTypeConversion  OutDataTypeStr=uint8
  Data Type Conversion1 : DataTypeConversion  OutDataTypeStr=uint16
  Data Type Conversion2 : DataTypeConversion  OutDataTypeStr=int32
  EtherCAT PDO Receive : xpcethercatlib/EtherCAT PDO Receive  Priority=2  sig_name=Box 4 (ATRIAS 2.1 Leg (Medulla 1.5)).Incremental Encoder.Incremental Encoder  sig_offset=992  sig_type=uint16  type_size=16  sig_dim=1  device_id=0  sample_time=0.001000
  EtherCAT PDO Receive1 : xpcethercatlib/EtherCAT PDO Receive  Priority=2  sig_name=Box 4 (ATRIAS 2.1 Leg (Medulla 1.5)).Incremental Encoder.Incremental Encoder Timestamp  sig_offset=1008  sig_type=uint16  type_size=16  sig_dim=1  device_id=0  sample_time=0.001000
  EtherCAT PDO Receive10 : xpcethercatlib/EtherCAT PDO Receive  Priority=2  sig_name=Box 4 (ATRIAS 2.1 Leg (Medulla 1.5)).Power.Logic Voltage  sig_offset=1040  sig_type=uint16  type_size=16  sig_dim=1  device_id=0  sample_time=0.001000
  EtherCAT PDO Receive11 : xpcethercatlib/EtherCAT PDO Receive  Priority=2  sig_name=Box 4 (ATRIAS 2.1 Leg (Medulla 1.5)).Power.Motor Voltage  sig_offset=1024  sig_type=uint16  type_size=16  sig_dim=1  device_id=0  sample_time=0.001000
  EtherCAT PDO Receive12 : xpcethercatlib/EtherCAT PDO Receive  Priority=2  sig_name=Box 4 (ATRIAS 2.1 Leg (Medulla 1.5)).Thermistors.Thermistor 0  sig_offset=1056  sig_type=uint16  type_size=16  sig_dim=1  device_id=0  sample_time=0.001000
  EtherCAT PDO Receive13 : xpcethercatlib/EtherCAT PDO Receive  Priority=2  sig_name=Box 4 (ATRIAS 2.1 Leg (Medulla 1.5)).Thermistors.Thermistor 1  sig_offset=1072  sig_type=uint16  type_size=16  sig_dim=1  device_id=0  sample_time=0.001000
  EtherCAT PDO Receive14 : xpcethercatlib/EtherCAT PDO Receive  Priority=2  sig_name=Box 4 (ATRIAS 2.1 Leg (Medulla 1.5)).Thermistors.Thermistor 2  sig_offset=1088  sig_type=uint16  type_size=16  sig_dim=1  device_id=0  sample_time=0.001000
  EtherCAT PDO Receive15 : xpcethercatlib/EtherCAT PDO Receive  Priority=2  sig_name=Box 4 (ATRIAS 2.1 Leg (Medulla 1.5)).Thermistors.Thermistor 3  sig_offset=1104  sig_type=uint16  type_size=16  sig_dim=1  device_id=0  sample_time=0.001000
  EtherCAT PDO Receive16 : xpcethercatlib/EtherCAT PDO Receive  Priority=2  sig_name=Box 4 (ATRIAS 2.1 Leg (Medulla 1.5)).Thermistors.Thermistor 4  sig_offset=1120  sig_type=uint16  type_size=16  sig_dim=1  device_id=0  sample_time=0.001000
  EtherCAT PDO Receive17 : xpcethercatlib/EtherCAT PDO Receive  Priority=2  sig_name=Box 4 (ATRIAS 2.1 Leg (Medulla 1.5)).Thermistors.Thermistor 5  sig_offset=1136  sig_type=uint16  type_size=16  sig_dim=1  device_id=0  sample_time=0.001000
  EtherCAT PDO Receive18 : xpcethercatlib/EtherCAT PDO Receive  Priority=2  sig_name=Box 4 (ATRIAS 2.1 Leg (Medulla 1.5)).uController Status.Counter  sig_offset=856  sig_type=uint8  type_size=8  sig_dim=1  device_id=0  sample_time=0.001000
  EtherCAT PDO Receive19 : xpcethercatlib/EtherCAT PDO Receive  Priority=2  sig_name=Box 4 (ATRIAS 2.1 Leg (Medulla 1.5)).uController Status.Error Flags  sig_offset=864  sig_type=uint8  type_size=8  sig_dim=1  device_id=0  sample_time=0.001000
  EtherCAT PDO Receive2 : xpcethercatlib/EtherCAT PDO Receive  Priority=2  sig_name=Box 4 (ATRIAS 2.1 Leg (Medulla 1.5)).Knee Force.Knee Force 1  sig_offset=1184  sig_type=uint16  type_size=16  sig_dim=1  device_id=0  sample_time=0.001000
  EtherCAT PDO Receive20 : xpcethercatlib/EtherCAT PDO Receive  Priority=2  sig_name=Box 4 (ATRIAS 2.1 Leg (Medulla 1.5)).uController Status.ID  sig_offset=840  sig_type=uint8  type_size=8  sig_dim=1  device_id=0  sample_time=0.001000
  EtherCAT PDO Receive21 : xpcethercatlib/EtherCAT PDO Receive  Priority=2  sig_name=Box 4 (ATRIAS 2.1 Leg (Medulla 1.5)).uController Status.State  sig_offset=848  sig_type=uint8  type_size=8  sig_dim=1  device_id=0  sample_time=0.001000
  EtherCAT PDO Receive22 : xpcethercatlib/EtherCAT PDO Receive  Priority=2  sig_name=Box 4 (ATRIAS 2.1 Leg (Medulla 1.5)).uController Status.Limit Switch  sig_offset=872  sig_type=uint8  type_size=8  sig_dim=1  device_id=0  sample_time=0.001000
  EtherCAT PDO Receive23 : xpcethercatlib/EtherCAT PDO Receive  Priority=2  sig_name=Box 4 (ATRIAS 2.1 Leg (Medulla 1.5)).uController Status.Toe Sensor  sig_offset=880  sig_type=uint16  type_size=16  sig_dim=1  device_id=0  sample_time=0.001000
  EtherCAT PDO Receive3 : xpcethercatlib/EtherCAT PDO Receive  Priority=2  sig_name=Box 4 (ATRIAS 2.1 Leg (Medulla 1.5)).Knee Force.Knee Force 2  sig_offset=1200  sig_type=uint16  type_size=16  sig_dim=1  device_id=0  sample_time=0.001000
  EtherCAT PDO Receive4 : xpcethercatlib/EtherCAT PDO Receive  Priority=2  sig_name=Box 4 (ATRIAS 2.1 Leg (Medulla 1.5)).Leg Encoder.Leg Encoder  sig_offset=944  sig_type=uint32  type_size=32  sig_dim=1  device_id=0  sample_time=0.001000
  EtherCAT PDO Receive5 : xpcethercatlib/EtherCAT PDO Receive  Priority=2  sig_name=Box 4 (ATRIAS 2.1 Leg (Medulla 1.5)).Leg Encoder.Leg Encoder Timestamp  sig_offset=976  sig_type=uint16  type_size=16  sig_dim=1  device_id=0  sample_time=0.001000
  EtherCAT PDO Receive6 : xpcethercatlib/EtherCAT PDO Receive  Priority=2  sig_name=Box 4 (ATRIAS 2.1 Leg (Medulla 1.5)).Measured Current.Amp 1 Measured Current  sig_offset=1152  sig_type=int16  type_size=16  sig_dim=1  device_id=0  sample_time=0.001000
  EtherCAT PDO Receive7 : xpcethercatlib/EtherCAT PDO Receive  Priority=2  sig_name=Box 4 (ATRIAS 2.1 Leg (Medulla 1.5)).Measured Current.Amp 2 Measured Current  sig_offset=1168  sig_type=int16  type_size=16  sig_dim=1  device_id=0  sample_time=0.001000
  EtherCAT PDO Receive8 : xpcethercatlib/EtherCAT PDO Receive  Priority=2  sig_name=Box 4 (ATRIAS 2.1 Leg (Medulla 1.5)).Motor Encoder.Motor Encoder  sig_offset=896  sig_type=uint32  type_size=32  sig_dim=1  device_id=0  sample_time=0.001000
  EtherCAT PDO Receive9 : xpcethercatlib/EtherCAT PDO Receive  Priority=2  sig_name=Box 4 (ATRIAS 2.1 Leg (Medulla 1.5)).Motor Encoder.Motor Encoder Timestamp  sig_offset=928  sig_type=uint16  type_size=16  sig_dim=1  device_id=0  sample_time=0.001000
  EtherCAT PDO Transmit : xpcethercatlib/EtherCAT PDO Transmit   Priority=3  sig_name=Box 4 (ATRIAS 2.1 Leg (Medulla 1.5)).uControllerInput.Command  sig_offset=840  sig_type=uint8  type_size=8  sig_dim=1  device_id=0  sample_time=0.001000
  EtherCAT PDO Transmit1 : xpcethercatlib/EtherCAT PDO Transmit   Priority=3  sig_name=Box 4 (ATRIAS 2.1 Leg (Medulla 1.5)).uControllerInput.Counter  sig_offset=848  sig_type=uint16  type_size=16  sig_dim=1  device_id=0  sample_time=0.001000
  EtherCAT PDO Transmit2 : xpcethercatlib/EtherCAT PDO Transmit   Priority=3  sig_name=Box 4 (ATRIAS 2.1 Leg (Medulla 1.5)).uControllerInput.Motor Current  sig_offset=864  sig_type=int32  type_size=32  sig_dim=1  device_id=0  sample_time=0.001000
  LegEncoder : Outport
  MotorEncoder : Outport  Port=2
  ToeSensor : Outport  Port=3
  LimitSwitch : Outport  Port=4
  ID : Outport  Port=5
  State : Outport  Port=6
  Counter : Outport  Port=7
  ErrorFlags : Outport  Port=8
  IncEncoder : Outport  Port=9
  LegEncoderTimestamp : Outport  Port=10
  MotorEncoderTimestamp : Outport  Port=11
  IncEncoderTimestamp : Outport  Port=12
  MotorVoltage : Outport  Port=13
  LogicVoltage : Outport  Port=14
  Thermistor0 : Outport  Port=15
  Thermistor1 : Outport  Port=16
  Thermistor2 : Outport  Port=17
  Thermistor3 : Outport  Port=18
  Thermistor4 : Outport  Port=19
  Thermistor5 : Outport  Port=20
  Amp1MeasuredCurrent : Outport  Port=21
  Amp2MeasuredCurrent : Outport  Port=22
  KneeForce1 : Outport  Port=23
  KneeForce2 : Outport  Port=24
  wires:
  Data Type Conversion/1 -> EtherCAT PDO Transmit/1
  Data Type Conversion1/1 -> EtherCAT PDO Transmit1/1
  Data Type Conversion2/1 -> EtherCAT PDO Transmit2/1
  EtherCAT PDO Receive/1 -> IncEncoder/1
  EtherCAT PDO Receive1/1 -> IncEncoderTimestamp/1
  EtherCAT PDO Receive2/1 -> KneeForce1/1
  EtherCAT PDO Receive3/1 -> KneeForce2/1
  EtherCAT PDO Receive4/1 -> LegEncoder/1
  EtherCAT PDO Receive5/1 -> LegEncoderTimestamp/1
  EtherCAT PDO Receive6/1 -> Amp1MeasuredCurrent/1
  EtherCAT PDO Receive7/1 -> Amp2MeasuredCurrent/1
  EtherCAT PDO Receive8/1 -> MotorEncoder/1
  EtherCAT PDO Receive9/1 -> MotorEncoderTimestamp/1
  EtherCAT PDO Receive10/1 -> LogicVoltage/1
  EtherCAT PDO Receive11/1 -> MotorVoltage/1
  EtherCAT PDO Receive12/1 -> Thermistor0/1
  EtherCAT PDO Receive13/1 -> Thermistor1/1
  EtherCAT PDO Receive14/1 -> Thermistor2/1
  EtherCAT PDO Receive15/1 -> Thermistor3/1
  EtherCAT PDO Receive16/1 -> Thermistor4/1
  EtherCAT PDO Receive17/1 -> Thermistor5/1
  EtherCAT PDO Receive18/1 -> Counter/1
  EtherCAT PDO Receive19/1 -> ErrorFlags/1
  EtherCAT PDO Receive20/1 -> ID/1
  EtherCAT PDO Receive22/1 -> LimitSwitch/1
  EtherCAT PDO Receive21/1 -> State/1
  EtherCAT PDO Receive23/1 -> ToeSensor/1
  MedullaCmd/1 -> Data Type Conversion/1
  MedullaCounter/1 -> Data Type Conversion1/1
  MotorCmd/1 -> Data Type Conversion2/1
